simulink model "Planner"  (R2020b)
settings: Solver=FixedStepAuto  StartTime=0.0  StopTime=11  FixedStep=0.001  RelTol=1e-3
values from neighbouring files (symbols this model uses):
  a0 = 0.99    [init.m]
  berta = 0.98    [init.m]
  csi = 1    [init.m]
  e_max = 0.01    [init.m]
  F_int_max = [2;2]    [init.m]
  F_max = [2;2]    [init.m]
  M = 0.1    [init.m]
  mass = 0.1    [init.m]
settings Model: Creator=chiara-s  LastModifiedBy=giorg

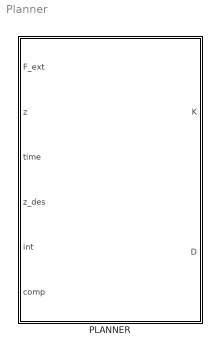
== system Planner ==
  PLANNER : Subsystem

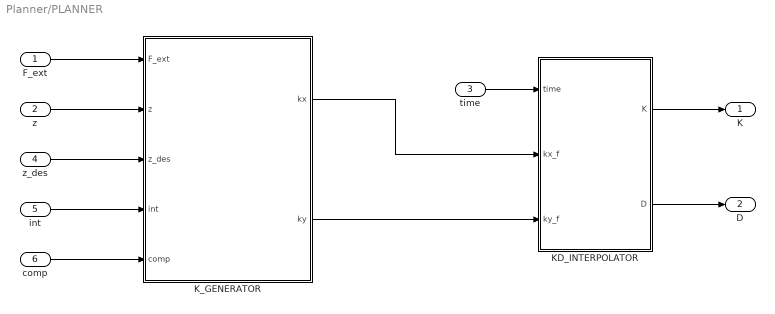
== system Planner/PLANNER ==
  F_ext : Inport
  z : Inport  Port=2
  time : Inport  Port=3
  z_des : Inport  Port=4
  int : Inport  Port=5
  comp : Inport  Port=6
  "KD_INTERPOLATOR " : MATLAB Function  TreatAsAtomicUnit=on
  K_GENERATOR : MATLAB Function  TreatAsAtomicUnit=on
  K : Outport
  D : Outport  Port=2
  wires:
  time/1 -> "KD_INTERPOLATOR "/1(time)
  "KD_INTERPOLATOR "/2(D) -> D/1
  "KD_INTERPOLATOR "/1(K) -> K/1
  K_GENERATOR/2(ky) -> "KD_INTERPOLATOR "/3(ky_f)
  K_GENERATOR/1(kx) -> "KD_INTERPOLATOR "/2(kx_f)
  int/1 -> K_GENERATOR/4(int)
  comp/1 -> K_GENERATOR/5(comp)
  F_ext/1 -> K_GENERATOR/1(F_ext)
  z/1 -> K_GENERATOR/2(z)
  z_des/1 -> K_GENERATOR/3(z_des)

== matlab function Planner/PLANNER/KD_INTERPOLATOR  ==
  settings: updateMethod=DISCRETE  sampleTime=Ts
  data: time input; K output; kx_f input; ky_f input; D output; e_max parameter; F_max parameter; M parameter; berta parameter; a0 parameter; mass parameter; csi parameter
function [K,D] = fcn(time, kx_f, ky_f, e_max, F_max, M, berta, a0, mass, csi)
%% Description
% Interpolate K in order to guarantee stability

%% Outputs
% K             Stiffness matrix
% D             Damping matrix

%% Inputs
% kx_f, ky, f   desired values of K

%% Parameters
% F_max         nominal disturbance forces
% e_max         maximum steady-state error
% M             virtual mass
% berta, a0     parameters for the computation of stability conditions
% mass          virtual mass

%% persistent initialization
persistent kx ky time_prec
if isempty(time_prec)
    time_prec = 0;              % previous simulation time
end
if isempty(kx)
   kx = F_max(1)/e_max;         % last value of k
end
if isempty(ky)
   ky = F_max(2)/e_max;
end

% set k from desired one 
if kx_f <= kx       
    kx = kx_f;
else 
    % increese k in accordance with the stability conditions
    kx_i = kx;
    k_dotx = berta*(4*a0*sqrt(kx_i/mass)*(kx_i)^(3/2))/(sqrt(kx_i) + 2*a0*csi*sqrt(kx_i));
    k_tempx = kx_i + k_dotx*(time -time_prec);
    if k_tempx > kx_f
        kx = kx_f;
    else
        kx = k_tempx;
    end
end

% Y axes, same as X axes
if ky_f <= ky
    ky = ky_f;
else 
    ky_i = ky;
    k_doty = berta*(4*a0*sqrt(ky_i/mass)*(ky_i)^(3/2))/(sqrt(ky_i) + 2*a0*csi*sqrt(ky_i));
    k_tempy = ky_i + k_doty*(time -time_prec);
    if k_tempy > ky_f
        ky = ky_f;
    else
        ky = k_tempy;
    end
end
time_prec = time;

% damping computation, critically damped condition
dx = sqrt(4*kx*M);
dy = sqrt(4*ky*M);

%% Final impedance matrices
D = diag([dx,dy]);
K = diag([kx,ky]);

end

== matlab function Planner/PLANNER/K_GENERATOR ==
  settings: updateMethod=DISCRETE  sampleTime=Ts
  data: kx output; F_ext input; z input; z_des input; int input; comp input; ky output; e_max parameter; F_max parameter; F_int_max parameter
function [kx, ky] = fcn(F_ext, z, z_des, int, comp, e_max, F_max, F_int_max)
%% Description
% Set the K coefficients for a variable impedance controller based on a
% desired trajectory

%% Outputs
% kx, ky            stiffness among axes

%% Inputs
% F_ext         measured external force
% z_des         desired trajectory
% z             current position
% int, comp     booleans for the interaction and compensation phase

%% Parameters
% F_int_max     desired interaction force
% F_max         nominal disturbance forces
% e_max         maximum steady-state error

%% persistent initialization
persistent kxi kyi kxc kyc F_comp int_prec comp_prec z_int z_int_dir 
if isempty(kxi)
   kxi = F_max(1)/e_max;        % k obtained from interaction
end
if isempty(kyi)
   kyi = F_max(2)/e_max;
end
if isempty(F_comp)
   F_comp = [0;0];              % weight to compensate
end
if isempty(kxc)
      kxc = F_max(1)/e_max;     % k obtained from compensation
end
if isempty(kyc)
      kyc = F_max(2)/e_max;
end
if isempty(z_int) 
    z_int = [1000; 1000];       % obstacle(or interaction) position
end
if isempty(z_int_dir) 
    z_int_dir = [0;0];          % prohibited direction due to the obstacle
end
if isempty(int_prec)
    int_prec = [0;0];           % previous values of int
end
if isempty(comp_prec)
    comp_prec = [0;0];          % previous values od comp
end

%% INTERACTION
% set kxi in order to match a desired interaction force with the
% envirorment, and store interaction's position when detected
% X axes
if int(1) == 1
    % detection of an interaction 
    if abs(F_ext(1)-F_comp(1)) > F_max(1)
        if z_int(1) == 1000                     % z_int has not been set yet
            z_int(1) = z(1);
            z_int_dir(1) = -sign(F_ext(1)-F_comp(1));
        end
    end
    % setting of kxi
    if abs(F_ext(1)-F_comp(1)) > F_int_max(1) 
        % if interaction force is higher than threshold
        if kxi*abs(z(1)-z_des(1)) > F_int_max(1)
            ktemp_x = F_int_max(1)/abs(z(1)-z_des(1));
            if ktemp_x < kxi                % kxi needs to be only decreased
                kxi = ktemp_x;
            end
        end
    end
end

% Y axes, same as X axes
if int(2) == 1
    if abs(F_ext(2)-F_comp(2)) > F_max(2)
        if z_int(2) == 1000
            z_int(2) = z(2);
            z_int_dir(2) = -sign(F_ext(2)-F_comp(2));
        end
    end
    if abs(F_ext(2)-F_comp(2)) > F_int_max(2) 
        if kyi*abs(z(2)-z_des(2)) > F_int_max(2)
            ktemp_y = F_int_max(2)/abs(z(2)-z_des(2));
            if ktemp_y < kyi
                kyi = ktemp_y;
            end
        end
    end
end

%% COMPENSATION
% set kxc in order to compensate the effect of the weight of the object,
% and store it
% X axes
if comp(1) == 1
    % compensation detection
    if z_int(1) == 1000                     % z_int not set before
       if abs(F_ext(1))/kxc > e_max         
            kxc = abs(F_ext(1))/e_max;
            F_comp(1) = F_ext(1);
       end
    else 
        if z_int_dir(1) == 1                % obstacle in above
            if z(1) < z_int(1)
                if abs(F_ext(1))/kxc > e_max 
                    kxc = abs(F_ext(1))/e_max;
                    F_comp(1) = F_ext(1);
                end
            end
        else                                % obstacle is below
            if z(1) > z_int(1)
                if abs(F_ext(1))/kxc > e_max
                    kxc = abs(F_ext(1))/e_max;
                    F_comp(1) = F_ext(1);
                end
            end
        end 
   end
end

% Y axes, same as X
if comp(2) == 1
    if z_int(2) == 1000 
       if abs(F_ext(2))/kyc > e_max
            kyc = abs(F_ext(2))/e_max;
            F_comp(2) = F_ext(2);
       end
    else 
        if z_int_dir(2) == 1
            if z(2) < z_int(2)
                if abs(F_ext(2))/kyc > e_max
                    kyc = abs(F_ext(2))/e_max;
                    F_comp(2) = F_ext(2);
                end
            end
        else
            if z(2) > z_int(2)
                if abs(F_ext(2))/kyc > e_max
                    kyc = abs(F_ext(2))/e_max;
                    F_comp(2) = F_ext(2);
                end
            end
        end  
   end
end

%% reset to default values when comp or int shifts to zero
if comp(1)==0 && comp_prec(1)==1
    kxc = F_max(1)/e_max;
    F_comp(1) = 0;
end
if comp(2)==0 && comp_prec(2)==1
    kyc = F_max(2)/e_max;
    F_comp(2) = 0;
end
if int(1)==0 && int_prec(1)==1
    kxi = F_max(1)/e_max;
end
if int(2)==0 && int_prec(2)==1
    kyi = F_max(2)/e_max;
end

%% from int to comp and vice versa
if int(1)==1 && int_prec(1)==0
    if comp_prec(1) == 1
        kxi = kxc;
    end
    z_int(1)=1000;
    z_int_dir(1)=0;
end
if int(2)==1 && int_prec(2)==0
    if comp_prec(2) == 1
        kyi = kyc;
    end
    z_int(2)=1000;
    z_int_dir(2)=0;
end
if comp(1) == 1 && comp_prec(1)==0
    if int_prec(1) == 1
        kxc = kxi;
    end
end
if comp(2) == 1 && comp_prec(2)==0
    if int_prec(2)==1
        kyc =kyi;
    end
end

% update to last booleans
int_prec = int;
comp_prec = comp;


%% Selection of Final Values of D-K
% default values
kx = abs(F_max(1))/e_max;
ky = abs(F_max(2))/e_max;

% compensation
if comp(1) == 1
    kx = kxc;
end
if comp(2) == 1
    ky = kyc;
end

% both compensation and interaction are activated
% if "away" from obstacle set kx = kxc else kxi
if int(1) == 1
    kx = kxi;
    if comp(1) == 1
        if z_int(1) == 1000
            kx = kxc;                       % obstacle not reached
        else
            if z_int_dir(1) == 1
                if z_des(1) < z_int(1)
                    kx = kxc;               % obstacle reached but "going away"
                end
            else
                if z_des(1) > z_int(1)
                    kx = kxc;               % obstacle reached but "going away"
                end
            end
        end
    else
        if z_int(1) == 1000
            kx = F_max(1)/e_max;            % restore to default
        else
            if z_int_dir(1) == 1
                if z_des(1) < z_int(1)
                    kx = F_max(1)/e_max;    % restore because "going away"
                end
            else
                if z_des(1) > z_int(1)
                    kx = F_max(1)/e_max;    % restore because "going away"
                end
            end
        end
    end
end

% sam as X
if int(2) == 1
    ky = kyi;
    if comp(2) == 1
        if z_int(2) == 1000
            kx = kxc;
        else
            if z_int_dir(2) == 1
                if z_des(2) < z_int(2) 
                    ky = kyc;
                end
            else
                if z_des(2) > z_int(2)
                    ky = kyc;
                end
            end
        end
    else
        if z_int(2) == 1000
            kx = F_max(2)/e_max;
        else
            if z_int_dir(2) == 1
                if z_des(2) < z_int(2) 
                    ky = F_max(2)/e_max;
                end
            else
                if z_des(2) > z_int(2)
                    ky = F_max(2)/e_max;
                end
            end
        end
    end
end

end
